simulink model "MDS_grasping"  (R2020b)
settings: Solver=FixedStepAuto  StartTime=0  StopTime=10.0  FixedStep=0.001  MaxStep=0.05  RelTol=1e-3
values from neighbouring files (symbols this model uses):
  e_max = 0.05    [init.m]
  F_max = [2;2]    [init.m]
  F_weight = [0;-50]    [init.m]
  M = 1    [init.m]
  mass = 1    [init.m]
settings Model: Creator=chiara-s  LastModifiedBy=chiara-s

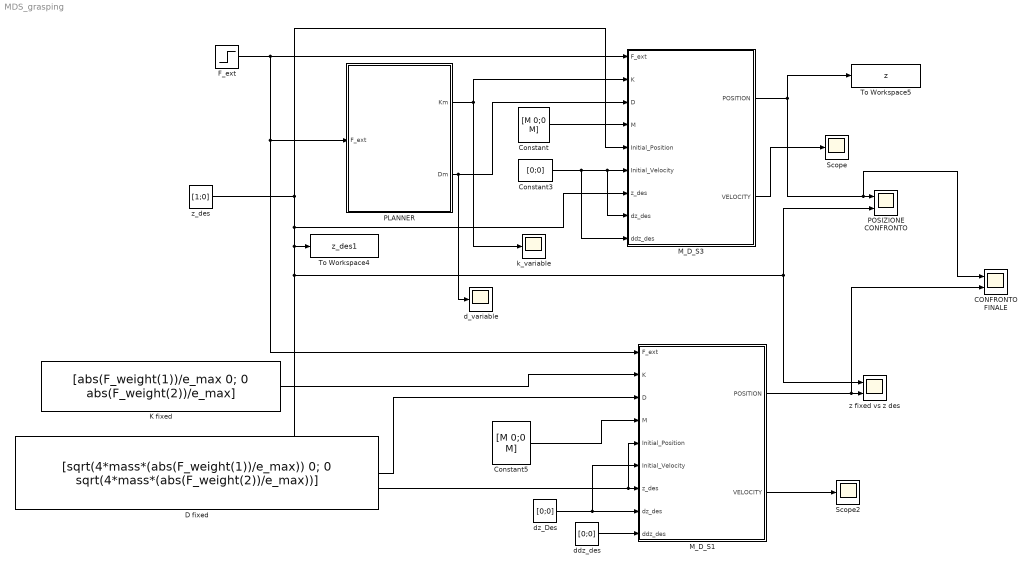
== system MDS_grasping ==
  CONFRONTO FINALE : Scope  NumInputPorts=2
  Constant : Constant  Value=[M 0;0 M]
  Constant3 : Constant  Value=[0;0]
  Constant5 : Constant  Value=[M 0;0 M]
  D fixed : Constant  Value=[sqrt(4*mass*(abs(F_weight(1))/e_max)) 0; 0 sqrt(4*mass*(abs(F_weight(2))/e_max))]
  F_ext : Step  Before=[0;0]  After=2*F_weight  SampleTime=0
  K fixed : Constant  Value=[abs(F_weight(1))/e_max 0; 0 abs(F_weight(2))/e_max]
  M_D_S1 : Subsystem
  M_D_S3 : Subsystem
  PLANNER : MATLAB Function  TreatAsAtomicUnit=on
  POSIZIONE CONFRONTO : Scope  NumInputPorts=2
  Scope : Scope
  Scope2 : Scope
  To Workspace4 : ToWorkspace  VariableName=z_des1  SaveFormat=Structure With Time  SampleTime=-1
      settings: Save2DSignal=2-D array (concatenate along first dimension)
  To Workspace5 : ToWorkspace  VariableName=z  SaveFormat=Structure With Time  SampleTime=-1
  d_variable : Scope
  ddz_des : Constant  Value=[0;0]
  dz_Des : Constant  Value=[0;0]
  k_variable : Scope
  z fixed vs z des : Scope  NumInputPorts=2
  z_des : Constant  Value=[1;0]
  wires:
  F_ext/1 -> M_D_S1/1(F_ext), PLANNER/1(F_ext), M_D_S3/1(F_ext)
  z_des/1 -> M_D_S3/5(Initial_Position), M_D_S1/5(Initial_Position), M_D_S1/7(z_des), z fixed vs z des/1, POSIZIONE CONFRONTO/2, To Workspace4/1, M_D_S3/7(z_des)
  PLANNER/1(Km) -> k_variable/1, M_D_S3/2(K)
  PLANNER/2(Dm) -> d_variable/1, M_D_S3/3(D)
  Constant/1 -> M_D_S3/4(M)
  Constant3/1 -> M_D_S3/6(Initial_Velocity), M_D_S3/8(dz_des), M_D_S3/9(ddz_des)
  M_D_S3/1(POSITION) -> To Workspace5/1, CONFRONTO FINALE/1, POSIZIONE CONFRONTO/1
  M_D_S3/2(VELOCITY) -> Scope/1
  dz_Des/1 -> M_D_S1/8(dz_des), M_D_S1/6(Initial_Velocity)
  ddz_des/1 -> M_D_S1/9(ddz_des)
  K fixed/1 -> M_D_S1/2(K)
  D fixed/1 -> M_D_S1/3(D)
  Constant5/1 -> M_D_S1/4(M)
  M_D_S1/2(VELOCITY) -> Scope2/1
  M_D_S1/1(POSITION) -> CONFRONTO FINALE/2, z fixed vs z des/2

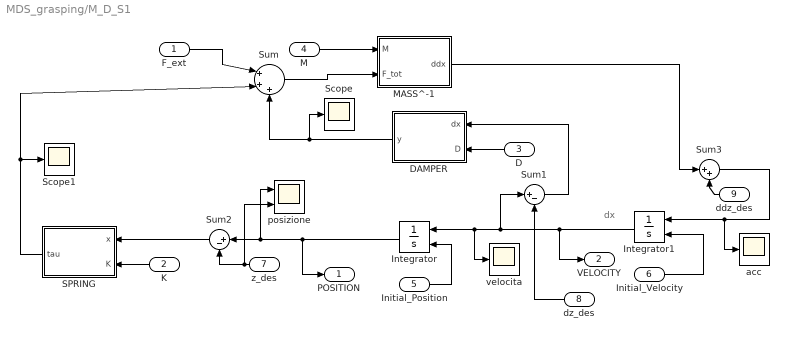
== system MDS_grasping/M_D_S1 ==
  note: dx
  F_ext : Inport
  K : Inport  Port=2
  D : Inport  Port=3
  M : Inport  Port=4
  Initial_Position : Inport  Port=5
  Initial_Velocity : Inport  Port=6
  z_des : Inport  Port=7
  dz_des : Inport  Port=8
  ddz_des : Inport  Port=9
  DAMPER : MATLAB Function  TreatAsAtomicUnit=on
  Integrator : Integrator  InitialConditionSource=external
  Integrator1 : Integrator  InitialConditionSource=external
  MASS^-1 : MATLAB Function  TreatAsAtomicUnit=on
  SPRING : MATLAB Function  TreatAsAtomicUnit=on
  Scope : Scope
  Scope1 : Scope
  Sum : Sum  Inputs=|+++
  Sum1 : Sum  Inputs=|+-
  Sum2 : Sum  Inputs=|+-
  Sum3 : Sum  Inputs=|++
  acc : Scope
  posizione : Scope  NumInputPorts=2
  velocita : Scope
  POSITION : Outport
  VELOCITY : Outport  Port=2
  wires:
  Integrator1/1 -> velocita/1, Integrator/1, Sum1/1, VELOCITY/1
  SPRING/1(tau) -> Sum/2, Scope1/1
  Integrator/1 -> posizione/1, Sum2/1, POSITION/1
  DAMPER/1(y) -> Scope/1, Sum/3
  Sum/1 -> MASS^-1/2(F_tot)
  M/1 -> MASS^-1/1(M)
  D/1 -> DAMPER/2(D)
  K/1 -> SPRING/2(K)
  Initial_Velocity/1 -> Integrator1/2
  Initial_Position/1 -> Integrator/2
  z_des/1 -> posizione/2, Sum2/2
  Sum2/1 -> SPRING/1(x)
  MASS^-1/1(ddx) -> Sum3/1
  Sum1/1 -> DAMPER/1(dx)
  Sum3/1 -> acc/1, Integrator1/1
  dz_des/1 -> Sum1/2
  ddz_des/1 -> Sum3/2
  F_ext/1 -> Sum/1

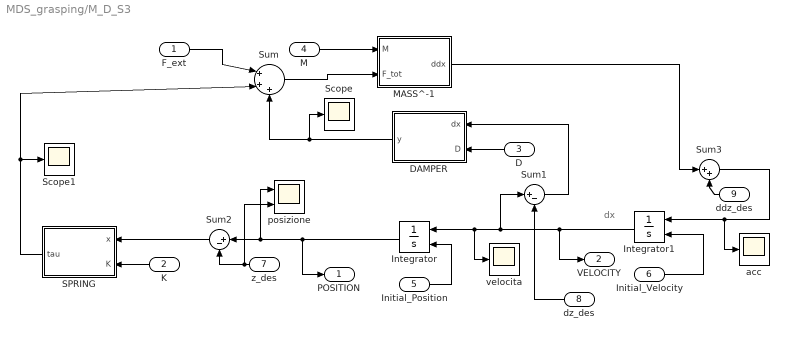
== system MDS_grasping/M_D_S3 ==
  note: dx
  F_ext : Inport
  K : Inport  Port=2
  D : Inport  Port=3
  M : Inport  Port=4
  Initial_Position : Inport  Port=5
  Initial_Velocity : Inport  Port=6
  z_des : Inport  Port=7
  dz_des : Inport  Port=8
  ddz_des : Inport  Port=9
  DAMPER : MATLAB Function  TreatAsAtomicUnit=on
  Integrator : Integrator  InitialConditionSource=external
  Integrator1 : Integrator  InitialConditionSource=external
  MASS^-1 : MATLAB Function  TreatAsAtomicUnit=on
  SPRING : MATLAB Function  TreatAsAtomicUnit=on
  Scope : Scope
  Scope1 : Scope
  Sum : Sum  Inputs=|+++
  Sum1 : Sum  Inputs=|+-
  Sum2 : Sum  Inputs=|+-
  Sum3 : Sum  Inputs=|++
  acc : Scope
  posizione : Scope  NumInputPorts=2
  velocita : Scope
  POSITION : Outport
  VELOCITY : Outport  Port=2
  wires:
  Integrator1/1 -> velocita/1, Integrator/1, Sum1/1, VELOCITY/1
  SPRING/1(tau) -> Sum/2, Scope1/1
  Integrator/1 -> posizione/1, Sum2/1, POSITION/1
  DAMPER/1(y) -> Scope/1, Sum/3
  Sum/1 -> MASS^-1/2(F_tot)
  M/1 -> MASS^-1/1(M)
  D/1 -> DAMPER/2(D)
  K/1 -> SPRING/2(K)
  Initial_Velocity/1 -> Integrator1/2
  Initial_Position/1 -> Integrator/2
  z_des/1 -> posizione/2, Sum2/2
  Sum2/1 -> SPRING/1(x)
  MASS^-1/1(ddx) -> Sum3/1
  Sum1/1 -> DAMPER/1(dx)
  Sum3/1 -> acc/1, Integrator1/1
  dz_des/1 -> Sum1/2
  ddz_des/1 -> Sum3/2
  F_ext/1 -> Sum/1

== matlab function MDS_grasping/M_D_S1/DAMPER ==
  data: dx input; y output; D input
function y = fcn(dx, D)
y = - D*dx;
end

== matlab function MDS_grasping/M_D_S1/MASS^-1 ==
  data: M input; ddx output; F_tot input
function ddx = fcn(M,F_tot)
ddx = (M^-1)*F_tot;
end

== matlab function MDS_grasping/M_D_S1/SPRING ==
  data: x input; tau output; K input
function tau = fcn(x, K)
tau= -K*x;
end

== matlab function MDS_grasping/M_D_S3/DAMPER ==
  data: dx input; y output; D input
function y = fcn(dx, D)
y = - D*dx;
end

== matlab function MDS_grasping/M_D_S3/MASS^-1 ==
  data: M input; ddx output; F_tot input
function ddx = fcn(M,F_tot)
ddx = (M^-1)*F_tot;
end

== matlab function MDS_grasping/M_D_S3/SPRING ==
  data: x input; tau output; K input
function tau = fcn(x, K)
tau= -K*x;
end

== matlab function MDS_grasping/PLANNER ==
  settings: updateMethod=DISCRETE  sampleTime=0.01
  data: Km output; Dm output; e_max parameter; F_max parameter; F_ext input; mass parameter; F_weight parameter
function [Km,Dm] = fcn(e_max, F_max, F_ext, mass, F_weight)

% with an estimated weight, k and d increase 
%% Outputs
% Km            stiffness matrix
% Dm            damping matrix 
%% Inputs
% time          current simulation time
% F_ext         measured external force

% variables initialization 
persistent kx ky dx dy
% initialization of k and d 
if isempty(kx)
   kx = max(F_max(1), abs(F_weight(1)))/e_max; 
end
if isempty(ky)
   ky = max(F_max(2), abs(F_weight(2)))/e_max;
end
if isempty(dx)
    dx = sqrt(4*kx*mass);
end
if isempty(dy)
    dy = sqrt(4*ky*mass);
end

% start algoritm with k variable
if abs(F_ext(1))/kx > e_max 
    kx = 1.02*kx;
    dx = sqrt(4*kx*mass);
end
if abs(F_ext(2))/ky > e_max
    ky = 1.02*ky;
    dy = sqrt(4*ky*mass);
end

% set k istantaneously
% kx = abs(F_ext(1))/e_max;
% ky = abs(F_ext(2))/e_max;

% Final Values of D-K
Dm = diag([dx,dy]);
Km = diag([kx,ky]);

end
